simulink model "chap13_1"  (Simulink 7.4)
settings: Solver=VariableStepDiscrete  StartTime=0.0  StopTime=10.0  RelTol=1e-3
settings Model: Creator=Administrator  LastModifiedBy=Administrator

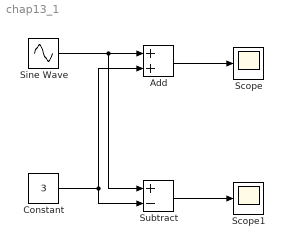
== system chap13_1 ==
  Add : Sum  OutDataType=fixdt(1, 16)  OutScaling=2^-10
  Constant : Constant  Value=3  OutDataType=fixdt(1, 16)  OutScaling=2^0
  Scope : Scope
  Scope1 : Scope
      settings: TickLabels=on
  Sine Wave : Sin  Amplitude=1  Bias=0  Frequency=5  Phase=0  Samples=10  SampleTime=0.01  Offset=0
  Subtract : Sum  Inputs=+-  OutDataType=fixdt(1, 16)  OutScaling=2^-10
  wires:
  Sine Wave/1 -> Add/1, Subtract/1
  Constant/1 -> Subtract/2, Add/2
  Add/1 -> Scope/1
  Subtract/1 -> Scope1/1
